simulink model "fxpdemo_sfun_user_dtprop"  (Simulink 7.6)
settings: Solver=FixedStepDiscrete  StartTime=0.0  StopTime=1  FixedStep=0.001  RelTol=1e-3
libraries: simulink x4
Description:
  | Fixed-Point S-Functions: Data Type Propagation
  | 
  | This model exercises a custom C language S-function written to enforce data types across multiple signals.
  | This operation is available in Simulink(R) with the "Data Type Propagation" block, which can be used for
  | comparison with this S-function example.
  | 
  | To see the source code for the S-function, use the right-click context menu to
  | select "Look Under Mask".  When the dialog box appears, press the Edit button.
settings Model: Creator=The MathWorks Inc.  ExtModeAutoUpdateStatusClock=off
settings DataIOCC: SignalLoggingName=sigsOut
settings OptimizationCC: InlineParams=on  InitFltsAndDblsToZero=on
settings DebuggingCC: SaveWithParameterizedLinksMsg=none  SignalResolutionControl=TryResolveAllWithWarning  SolverPrmCheckMsg=none  MultiTaskDSMMsg=warning  MultiTaskCondExecSysMsg=none  ParameterOverflowMsg=warning  ParameterPrecisionLossMsg=none  StrictBusMsg=None
settings HardwareCC: TargetUnknown=on
settings RTWCC: GenerateReport=on  IncludeERTFirstTime=on
settings GRTTargetCC: TargetFcnLib=ansi_tfl_tmw.mat

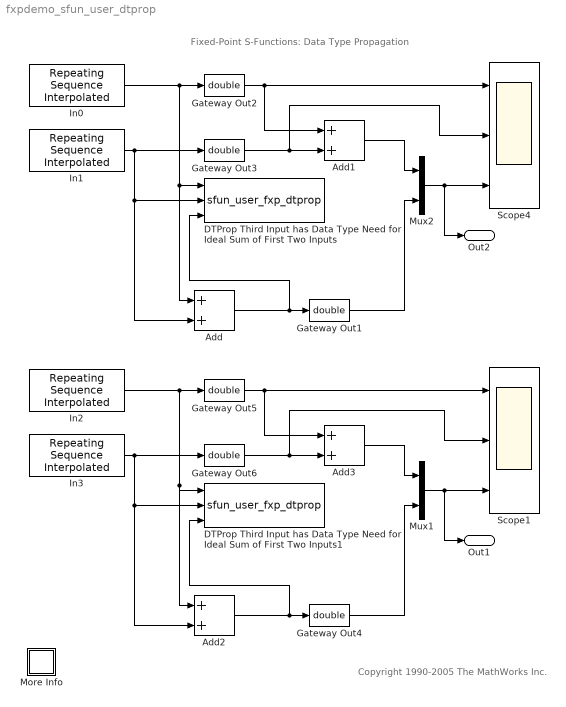
== system fxpdemo_sfun_user_dtprop ==
  note: Copyright 1990-2005 The MathWorks Inc.
  note: Fixed-Point S-Functions: Data Type Propagation
  Add : Sum  OutDataTypeStr=Inherit: Inherit via back propagation
  Add1 : Sum  OutDataTypeStr=double
  Add2 : Sum  OutDataTypeStr=Inherit: Inherit via back propagation
  Add3 : Sum  OutDataTypeStr=double
  DTProp Third Input has Data Type Need for Ideal Sum of First Two Inputs : S-Function  FunctionName=sfun_user_fxp_dtprop  EnableBusSupport=off
  DTProp Third Input has Data Type Need for Ideal Sum of First Two Inputs1 : S-Function  FunctionName=sfun_user_fxp_dtprop  EnableBusSupport=off
  Gateway Out{1..6} (6 alike) : DataTypeConversion  OutDataTypeStr=double  RndMeth=Zero
  In0 : simulink/Sources/Repeating Sequence Interpolated  SystemSampleTime=-1  OutValues=2^(16-1-8)*[-1 linspace(-1,0,5) 0 linspace(0,1,5) 1]  TimeValues=1/13*linspace(0,1,13)  LookUpMeth=Interpolation-Use End Values  tsamp=0.001  OutMin=[]  OutMax=[]  OutDataTypeStr=fixdt(1,16,8)  OutputDataTypeScalingMode=Specify via dialog  OutDataType=sfix(16)  OutScaling=2^-8
  In1 : simulink/Sources/Repeating Sequence Interpolated  SystemSampleTime=-1  OutValues=2^(16-1+(-5))*[-1 linspace(-1,0,5) 0 linspace(0,1,5) 1]  TimeValues=linspace(0,1,13)  LookUpMeth=Interpolation-Use End Values  tsamp=0.001  OutMin=[]  OutMax=[]  OutDataTypeStr=fixdt(1,16,5)  OutputDataTypeScalingMode=Specify via dialog  OutDataType=sfix(16)  OutScaling=2^-5
  In2 : simulink/Sources/Repeating Sequence Interpolated  SystemSampleTime=-1  OutValues=2^(5+(0))*[0 linspace(0,1,5) 1]  TimeValues=linspace(0,1,7)  LookUpMeth=Interpolation-Use End Values  tsamp=0.001  OutMin=[]  OutMax=[]  OutDataTypeStr=fixdt(0,5,0)  OutputDataTypeScalingMode=Specify via dialog  OutDataType=ufix(5)  OutScaling=2^0
  In3 : simulink/Sources/Repeating Sequence Interpolated  SystemSampleTime=-1  OutValues=2^(4+(-4))*[0 linspace(0,1,5) 1]  TimeValues=1/7*linspace(0,1,7)  LookUpMeth=Interpolation-Use End Values  tsamp=0.001  OutMin=[]  OutMax=[]  OutDataTypeStr=fixdt(0,4,4)  OutputDataTypeScalingMode=Specify via dialog  OutDataType=ufix(4)  OutScaling=2^-4
  More Info : Subsystem
      settings: OpenFcn=showdemo(bdroot(gcs))
      mask Display: disp('?')
  Mux1 : Mux  Inputs=2
  Mux2 : Mux  Inputs=2
  Scope1 : Scope  NumInputPorts=3
      settings: TimeRange=1  YMin=0~0~0  YMax=35~1~35
  Scope4 : Scope  NumInputPorts=3
      settings: TimeRange=1  YMin=-150~-1500~-1500  YMax=150~1500~1500  SaveName=ScopeData3
  Out2 : Outport
  Out1 : Outport  Port=2
  wires:
  In1/1 -> Add/2, DTProp Third Input has Data Type Need for Ideal Sum of First Two Inputs/2, Gateway Out3/1
  Add/1 -> DTProp Third Input has Data Type Need for Ideal Sum of First Two Inputs/3, Gateway Out1/1
  Add1/1 -> Mux2/1
  Mux2/1 -> Scope4/3, Out2/1
  In0/1 -> Gateway Out2/1, DTProp Third Input has Data Type Need for Ideal Sum of First Two Inputs/1, Add/1
  Gateway Out3/1 -> Add1/2, Scope4/2
  Gateway Out2/1 -> Add1/1, Scope4/1
  Gateway Out1/1 -> Mux2/2
  In3/1 -> Gateway Out6/1, DTProp Third Input has Data Type Need for Ideal Sum of First Two Inputs1/2, Add2/2
  Add2/1 -> Gateway Out4/1, DTProp Third Input has Data Type Need for Ideal Sum of First Two Inputs1/3
  Add3/1 -> Mux1/1
  Mux1/1 -> Out1/1, Scope1/3
  In2/1 -> Add2/1, DTProp Third Input has Data Type Need for Ideal Sum of First Two Inputs1/1, Gateway Out5/1
  Gateway Out6/1 -> Scope1/2, Add3/2
  Gateway Out5/1 -> Scope1/1, Add3/1
  Gateway Out4/1 -> Mux1/2

== system fxpdemo_sfun_user_dtprop/More Info ==
